simulink model "pvpanelPaper_2_5"  (R2020a)
settings: Solver=VariableStepAuto  StartTime=0.0  StopTime=10.0  RelTol=1e-3
settings Model: Creator=shrad  LastModifiedBy=shrad

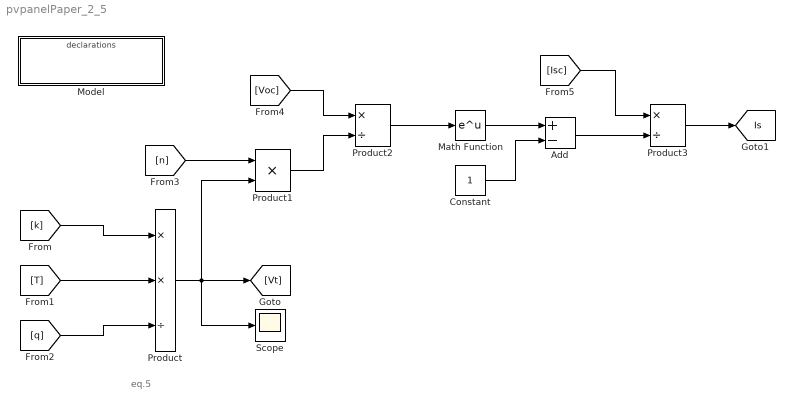
== system pvpanelPaper_2_5 ==
  note: eq.5
  Add : Sum  Inputs=+-
  Constant : Constant
  Math Function : Math  SaturateOnIntegerOverflow=on
  Model : ModelReference  ModelNameDialog=declarations.slx  SimulationMode=Normal  ModelReferenceVersion=1.2
  Product : Product  Inputs=**/
  Product1 : Product
  Product2 : Product  Inputs=*/
  Product3 : Product  Inputs=*/
  Scope : Scope
  tag scope: Is=global
  wires:
  [k] -> Product/1
  [T] -> Product/2
  [q] -> Product/3
  Product/1 -> Product1/2, Scope/1, [Vt]
  [n] -> Product1/1
  [Voc] -> Product2/1
  Product1/1 -> Product2/2
  Product2/1 -> Math Function/1
  Math Function/1 -> Add/1
  Constant/1 -> Add/2
  Add/1 -> Product3/2
  [Isc] -> Product3/1
  Product3/1 -> [Is]
